simulink model "simple_pwm_model"  (R2017a)
settings: Solver=VariableStepAuto  StartTime=0.0  StopTime=3  RelTol=1e-3
undefined symbols (not defined in the file or in its folder): clk
libraries: simulink x1
settings Model: Creator=mini  LastModifiedBy=mini
settings OptimizationCC: BlockReduction=off  ConditionallyExecuteInputs=off  DefaultParameterBehavior=Inlined
settings DebuggingCC: AlgebraicLoopMsg=error
settings HardwareCC: ProdBitPerPointer=32  ProdBitPerSizeT=32  ProdBitPerPtrDiffT=32  ProdLargestAtomicFloat=None  ProdIntDivRoundTo=Undefined  ProdEndianess=Unspecified  ProdWordSize=32  ProdHWDeviceType=ASIC/FPGA->ASIC/FPGA  ProdEqTarget=off

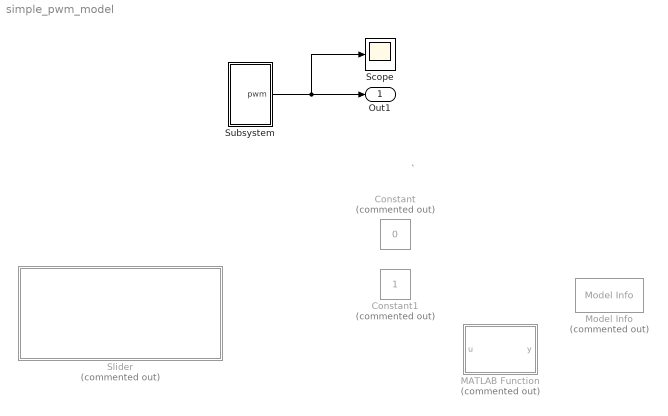
== system simple_pwm_model ==
  note: `
  Constant : Constant  Commented=on  Value=0
  Constant1 : Constant  Commented=on
  MATLAB Function : MATLAB Function  Commented=on  TreatAsAtomicUnit=on
  Model Info : simulink/Model-Wide Utilities/Model Info  Commented=on  Frame=on  DisplayStringWithTags=Model Info  HorizontalTextAlignment=Center  LeftAlignmentValue=0.5  SourceBlockDiagram=simulink  TagMaxNumber=20  mask(CMBlock){}
      mask DialogControl HERE Prompt: Hello
  Scope : Scope
  Slider : Subsystem  Commented=on  DialogController=hmiCreateDDGDialog  IsWebBlock=on  mask(MWDashboardBlock){webBlockId=13ed27be-1b6a-494e-91e5-f38899f76198, webBlockType=slider, ShowInLibBrowser=on, ShowInitialText=on, HMISrcModelName=simple_pwm_model}
      mask prompts: webBlockId "WebBlock Id"; webBlockType "WebBlock Type"; HMISrcModelName "Source Model"
      mask help: SimulinkHMI:dialogs:SliderDialogDesc
      mask Help: helpview([docroot '/mapfiles/simulink.map'], 'hmi_slider')
      mask Display:
      | if strcmp(get_param(bdroot(gcb),'BlockDiagramType'), 'library')
      |     image([(matlabroot) '/toolbox/simulink/hmi/icons/Slider.png']);
      | end
  Subsystem : Subsystem  TreatAsAtomicUnit=on
  Out1 : Outport  OutDataTypeStr=boolean
  wires:
  Subsystem/1(pwm) -> Scope/1, Out1/1

== system simple_pwm_model/Slider ==

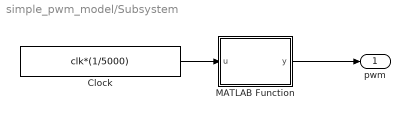
== system simple_pwm_model/Subsystem ==
  "Clock " : Constant  Value=clk*(1/5000)  OutDataTypeStr=uint32
  MATLAB Function : MATLAB Function  TreatAsAtomicUnit=on
  pwm : Outport
  wires:
  "Clock "/1 -> MATLAB Function/1(u)
  MATLAB Function/1(y) -> pwm/1

== matlab function simple_pwm_model/Subsystem/MATLAB Function ==
  data: u input; y output
function y = fcn(u)
    % generate PWM signal from clk
    if (u ~= previousInput)
        if (count > 100)
            count = 0;
        end
        count += 1;
        if (count < dutyCycle)
            output = 1;
        end
        previousInput = u;
    else
        output = previousOuptut;
    end
y = output;

== matlab function simple_pwm_model/MATLAB Function ==
  data: u input; y output
function y = fcn(u)
    y = u
